simulink model "thrust"  (Simulink 7.5)
settings: Solver=ode45  StartTime=0.0  StopTime=10.0  RelTol=1e-3
values from neighbouring files (symbols this model uses):
  Xs = 12.5    [valuables.m]
  YL = 0.6    [valuables.m]
  Zs = 0.25    [valuables.m]
undefined symbols (not defined in the file or in its folder): Xl, Zl
settings Model: Creator=knightofaccess  LastModifiedBy=knightofaccess

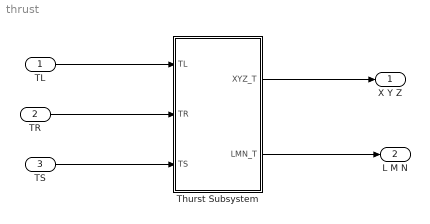
== system thrust ==
  TL : Inport  OutDataType=sfix(16)  OutScaling=2^0
  TR : Inport  Port=2  OutDataType=sfix(16)  OutScaling=2^0
  TS : Inport  Port=3  OutDataType=sfix(16)  OutScaling=2^0
  Thurst Subsystem : Subsystem
  X Y Z : Outport  OutDataType=sfix(16)  OutScaling=2^0
  L M N : Outport  Port=2  OutDataType=sfix(16)  OutScaling=2^0
  wires:
  Thurst Subsystem/1(XYZ_T) -> X Y Z/1
  Thurst Subsystem/2(LMN_T) -> L M N/1
  TL/1 -> Thurst Subsystem/1(TL)
  TR/1 -> Thurst Subsystem/2(TR)
  TS/1 -> Thurst Subsystem/3(TS)

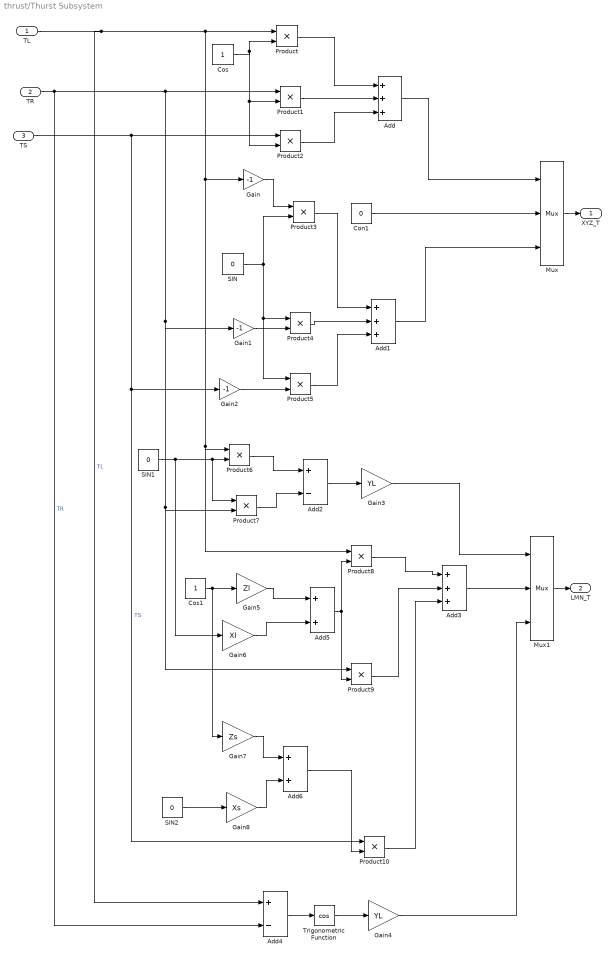
== system thrust/Thurst Subsystem ==
  TL : Inport  OutDataType=sfix(16)  OutScaling=2^0
  TR : Inport  Port=2  OutDataType=sfix(16)  OutScaling=2^0
  TS : Inport  Port=3  OutDataType=sfix(16)  OutScaling=2^0
  Add : Sum  Inputs=+++  OutDataType=sfix(16)  OutScaling=2^-10
  Add1 : Sum  Inputs=+++  OutDataType=sfix(16)  OutScaling=2^-10
  Add2 : Sum  Inputs=+-  OutDataType=sfix(16)  OutScaling=2^-10
  Add3 : Sum  Inputs=+++  OutDataType=sfix(16)  OutScaling=2^-10
  Add4 : Sum  Inputs=+-  OutDataType=sfix(16)  OutScaling=2^-10
  Add5 : Sum  OutDataType=sfix(16)  OutScaling=2^-10
  Add6 : Sum  OutDataType=sfix(16)  OutScaling=2^-10
  Con1 : Constant  Value=0  OutDataType=sfix(16)  OutScaling=2^0
  Cos : Constant  OutDataType=sfix(16)  OutScaling=2^0
  Cos1 : Constant  OutDataType=sfix(16)  OutScaling=2^0
  Gain : Gain  Gain=-1  ParameterDataType=sfix(16)  ParameterScaling=2^0  OutDataType=sfix(16)  OutScaling=2^0
  Gain1 : Gain  Gain=-1  ParameterDataType=sfix(16)  ParameterScaling=2^0  OutDataType=sfix(16)  OutScaling=2^0
  Gain2 : Gain  Gain=-1  ParameterDataType=sfix(16)  ParameterScaling=2^0  OutDataType=sfix(16)  OutScaling=2^0
  Gain3 : Gain  Gain=YL  ParameterDataType=sfix(16)  ParameterScaling=2^0  OutDataType=sfix(16)  OutScaling=2^0
  Gain4 : Gain  Gain=YL  ParameterDataType=sfix(16)  ParameterScaling=2^0  OutDataType=sfix(16)  OutScaling=2^0
  Gain5 : Gain  Gain=Zl  ParameterDataType=sfix(16)  ParameterScaling=2^0  OutDataType=sfix(16)  OutScaling=2^0
  Gain6 : Gain  Gain=Xl  ParameterDataType=sfix(16)  ParameterScaling=2^0  OutDataType=sfix(16)  OutScaling=2^0
  Gain7 : Gain  Gain=Zs  ParameterDataType=sfix(16)  ParameterScaling=2^0  OutDataType=sfix(16)  OutScaling=2^0
  Gain8 : Gain  Gain=Xs  ParameterDataType=sfix(16)  ParameterScaling=2^0  OutDataType=sfix(16)  OutScaling=2^0
  Mux : Mux  Inputs=3
  Mux1 : Mux  Inputs=3
  Product{,1..10} (11 alike) : Product  OutDataType=sfix(16)  OutScaling=2^0  RndMeth=Zero
  SIN : Constant  Value=0  OutDataType=sfix(16)  OutScaling=2^0
  SIN1 : Constant  Value=0  OutDataType=sfix(16)  OutScaling=2^0
  SIN2 : Constant  Value=0  OutDataType=sfix(16)  OutScaling=2^0
  Trigonometric Function : Trigonometry  Operator=cos  SampleTime=0
  XYZ_T : Outport  OutDataType=sfix(16)  OutScaling=2^0
  LMN_T : Outport  Port=2  OutDataType=sfix(16)  OutScaling=2^0
  wires:
  TL/1 -> Product/1, Gain/1, Product6/1, Product8/1, Add4/1  "TL"
  Cos/1 -> Product/2, Product1/2, Product2/2
  TR/1 -> Product1/1, Gain1/1, Product7/2, Product9/1, Add4/2  "TR"
  TS/1 -> Product2/1, Gain2/1, Product10/1  "TS"
  Product/1 -> Add/1
  Product1/1 -> Add/2
  Product2/1 -> Add/3
  SIN/1 -> Product3/2, Product4/1, Product5/1
  Gain/1 -> Product3/1
  Gain1/1 -> Product4/2
  Gain2/1 -> Product5/2
  Product3/1 -> Add1/1
  Product4/1 -> Add1/2
  Product5/1 -> Add1/3
  Add/1 -> Mux/1
  Con1/1 -> Mux/2
  Add1/1 -> Mux/3
  SIN1/1 -> Product6/2, Product7/1, Gain6/1
  Product6/1 -> Add2/1
  Product7/1 -> Add2/2
  Add2/1 -> Gain3/1
  Gain3/1 -> Mux1/1
  Product8/1 -> Add3/1
  Product9/1 -> Add3/2
  Product10/1 -> Add3/3
  Add3/1 -> Mux1/2
  Gain4/1 -> Mux1/3
  Mux/1 -> XYZ_T/1
  Mux1/1 -> LMN_T/1
  Gain5/1 -> Add5/1
  Cos1/1 -> Gain5/1, Gain7/1
  Gain6/1 -> Add5/2
  Add5/1 -> Product8/2, Product9/2
  SIN2/1 -> Gain8/1
  Gain7/1 -> Add6/1
  Gain8/1 -> Add6/2
  Add6/1 -> Product10/2
  Trigonometric Function/1 -> Gain4/1
  Add4/1 -> Trigonometric Function/1
